simulink model "P_k_calc"  (R2022a)
settings: Solver=VariableStepAuto  StartTime=0.0  StopTime=2  RelTol=1e-3
values from neighbouring files (symbols this model uses):
  A_DT = SS_DT.A    [TestDiscreteTimeSimulink.m]
  B_DT = SS_DT.B    [TestDiscreteTimeSimulink.m]
  C = [0 0 1]    [DAE_Circuit_main.m]    (also in SimulinkInput.mat = [1  0  0; 0  1  0; 0  0  1]; Test.mat = [1 0 0]; TestDiscreteTimeSimulink.m = [1 0)
  Q = SIM.Q_0*eye(N.inputs)    [DAE_Circuit_main.m]    (also in SimulinkInput.mat = 0.0001; Test.mat = 0.01; TestDiscreteTimeSimulink.m = Q_0*eye(N_inputs); TestSimulinkNoise_script.m = 0.0001)
  R = SIM.R_0*eye(N.measur)    [DAE_Circuit_main.m]    (also in SimulinkInput.mat = 0.0001; Test.mat = 0.0001; TestDiscreteTimeSimulink.m = R_0*eye(N_meas))
settings Model: Creator=tyevans  LastModifiedBy=tyevans

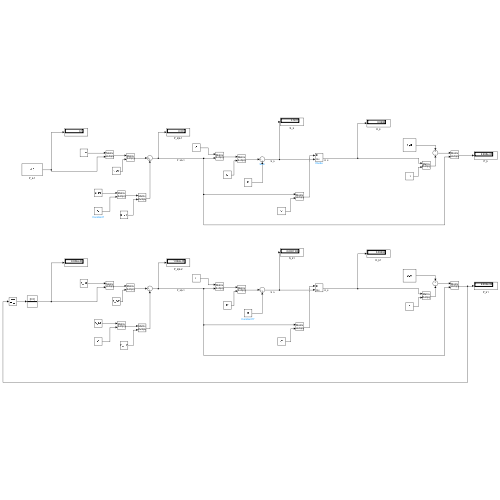
[thumbnail: Simulink's stored preview of the top-level diagram]
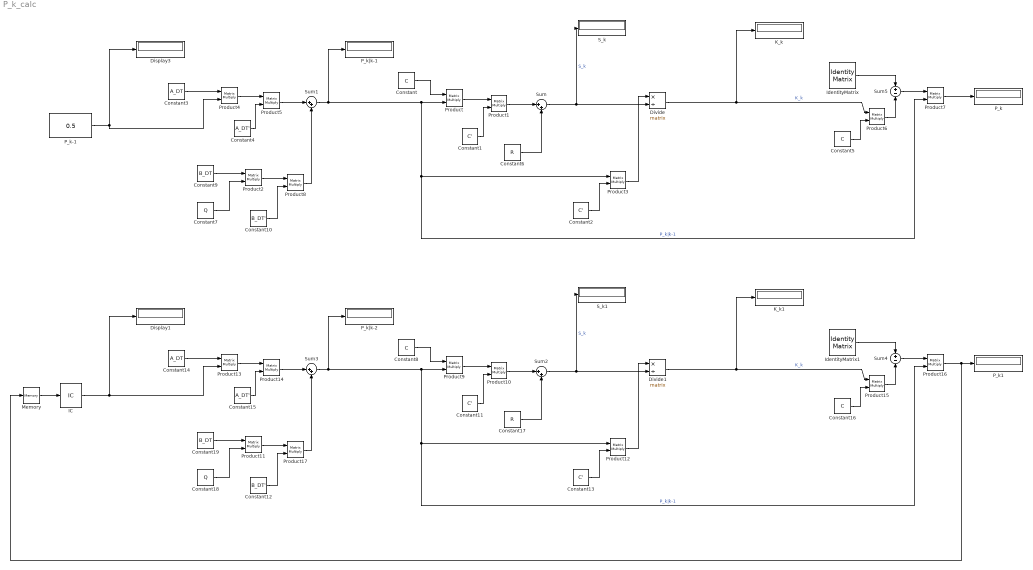
== system P_k_calc ==
  Constant{,5,8,16} (4 alike) : Constant  Value=C  VectorParams1D=off
  Constant{1..2,11,13} (4 alike) : Constant  Value=C'  VectorParams1D=off
  Constant10 : Constant  Value=B_DT'
  Constant12 : Constant  Value=B_DT'
  Constant14 : Constant  Value=A_DT  VectorParams1D=off
  Constant15 : Constant  Value=A_DT'  VectorParams1D=off
  Constant17 : Constant  Value=R
  Constant18 : Constant  Value=Q
  Constant19 : Constant  Value=B_DT
  Constant3 : Constant  Value=A_DT  VectorParams1D=off
  Constant4 : Constant  Value=A_DT'  VectorParams1D=off
  Constant6 : Constant  Value=R
  Constant7 : Constant  Value=Q
  Constant9 : Constant  Value=B_DT
  Display1 : Display
  Display3 : Display
  Divide : Product  Inputs=*/  Multiplication=Matrix(*)
  Divide1 : Product  Inputs=*/  Multiplication=Matrix(*)
  IC : InitialCondition  Value=0.5
  IdentityMatrix : IdentityMatrix  OutputDimensions=N_states  SampleTime=-1
  IdentityMatrix1 : IdentityMatrix  OutputDimensions=N_states  SampleTime=-1
  K_k : Display
  K_k1 : Display
  Memory : Memory
  P_k : Display
  P_k-1 : Constant  Value=0.5
  P_k1 : Display
  P_k|k-1 : Display
  P_k|k-2 : Display
  Product{,1..17} (18 alike) : Product  Multiplication=Matrix(*)
  S_k : Display
  S_k1 : Display
  Sum{,1..3} (4 alike) : Sum  Inputs=|++
  Sum4 : Sum  Inputs=+-
  Sum5 : Sum  Inputs=+-
  wires:
  Constant3/1 -> Product4/1
  Product4/1 -> Product5/1
  Constant4/1 -> Product5/2
  Constant/1 -> Product/1
  Product/1 -> Product1/1
  Constant1/1 -> Product1/2
  Constant2/1 -> Product3/2
  Product3/1 -> Divide/1
  Divide/1 -> Product6/1, K_k/1  "K_k"
  P_k-1/1 -> Product4/2, Display3/1
  Product1/1 -> Sum/1
  Constant6/1 -> Sum/2
  Sum/1 -> Divide/2, S_k/1  "S_k"
  Product5/1 -> Sum1/1
  Sum1/1 -> Product3/1, Product7/2, Product/2, P_k|k-1/1  "P_k|k-1"
  Constant9/1 -> Product2/1
  Constant7/1 -> Product2/2
  Product2/1 -> Product8/1
  Constant10/1 -> Product8/2
  Product8/1 -> Sum1/2
  Constant5/1 -> Product6/2
  Product6/1 -> Sum5/2
  IdentityMatrix/1 -> Sum5/1
  Sum5/1 -> Product7/1
  Product7/1 -> P_k/1
  Memory/1 -> IC/1
  Constant12/1 -> Product17/2
  Constant15/1 -> Product14/2
  Sum2/1 -> Divide1/2, S_k1/1  "S_k"
  Product12/1 -> Divide1/1
  Constant14/1 -> Product13/1
  Divide1/1 -> Product15/1, K_k1/1  "K_k"
  Constant13/1 -> Product12/2
  Product9/1 -> Product10/1
  Product14/1 -> Sum3/1
  Sum3/1 -> Product12/1, Product16/2, Product9/2, P_k|k-2/1  "P_k|k-1"
  Constant18/1 -> Product11/2
  Constant11/1 -> Product10/2
  Constant19/1 -> Product11/1
  Product11/1 -> Product17/1
  Product13/1 -> Product14/1
  Product10/1 -> Sum2/1
  Constant16/1 -> Product15/2
  Sum4/1 -> Product16/1
  Product16/1 -> Memory/1, P_k1/1
  Product15/1 -> Sum4/2
  Constant8/1 -> Product9/1
  IdentityMatrix1/1 -> Sum4/1
  Product17/1 -> Sum3/2
  Constant17/1 -> Sum2/2
  IC/1 -> Product13/2, Display1/1
